simulink model "sim_quadrotor_16b"  (R2016b)
settings: Solver=ode4  StartTime=0.0  StopTime=20  FixedStep=0.0001  RelTol=1e-3
undefined symbols (not defined in the file or in its folder): Ag_phi_rad, Ag_psi_rad, Ag_theta_rad, AgVel_p_radPerScnd, AgVel_q_radPerScnd, AgVel_r_radPerScnd, Ap, Aq, Ar, Az, Bp, Bq, Br, Bz, C, D, par, Pos_z_mtr, V_w_mtrPerScnd
settings Model: Creator=Nu  LastModifiedBy=Nu

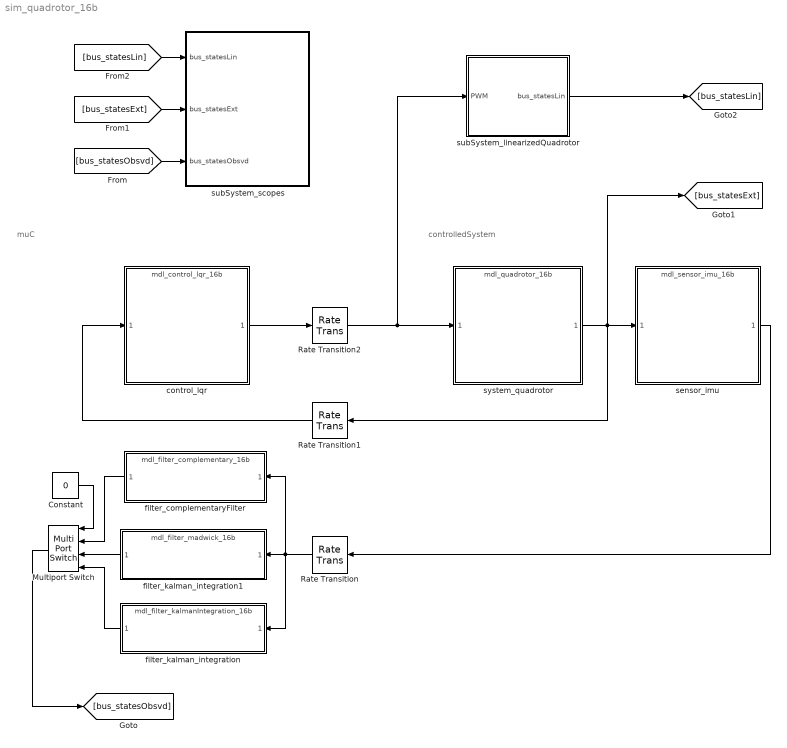
== system sim_quadrotor_16b ==
  note: controlledSystem
  note: muC
  Constant : Constant  Value=0
  Multiport Switch : MultiPortSwitch  DataPortOrder=Zero-based contiguous
  Rate Transition : RateTransition  OutPortSampleTime=filterKalman_par.T
  Rate Transition1 : RateTransition
  Rate Transition2 : RateTransition
  control_lqr : ModelReference  ModelNameDialog=mdl_control_lqr_16b.slx  SimulationMode=Normal  ModelReferenceVersion=1.230
  filter_complementaryFilter : ModelReference  ModelNameDialog=mdl_filter_complementary_16b.slx  SimulationMode=Normal  ModelReferenceVersion=1.30
  filter_kalman_integration : ModelReference  ModelNameDialog=mdl_filter_kalmanIntegration_16b.slx  SimulationMode=Normal  ModelReferenceVersion=1.24
  filter_kalman_integration1 : ModelReference  ModelNameDialog=mdl_filter_madwick_16b.slx  SimulationMode=Normal  ModelReferenceVersion=1.24
  sensor_imu : ModelReference  ModelNameDialog=mdl_sensor_imu_16b.slx  SimulationMode=Normal  ModelReferenceVersion=1.231
  subSystem_linearizedQuadrotor : Subsystem
  subSystem_scopes : Subsystem
  system_quadrotor : ModelReference  ModelNameDialog=mdl_quadrotor_16b.slx  SimulationMode=Normal  ModelReferenceVersion=1.231
  wires:
  system_quadrotor/1 -> Rate Transition1/1, sensor_imu/1, [bus_statesExt]
  control_lqr/1 -> Rate Transition2/1
  sensor_imu/1 -> Rate Transition/1
  [bus_statesObsvd] -> subSystem_scopes/3(bus_statesObsvd)
  [bus_statesExt] -> subSystem_scopes/2(bus_statesExt)
  [bus_statesLin] -> subSystem_scopes/1(bus_statesLin)
  subSystem_linearizedQuadrotor/1(bus_statesLin) -> [bus_statesLin]
  Rate Transition2/1 -> system_quadrotor/1, subSystem_linearizedQuadrotor/1(PWM)
  Multiport Switch/1 -> [bus_statesObsvd]
  Rate Transition/1 -> filter_kalman_integration1/1, filter_complementaryFilter/1, filter_kalman_integration/1
  Rate Transition1/1 -> control_lqr/1
  filter_complementaryFilter/1 -> Multiport Switch/2
  filter_kalman_integration/1 -> Multiport Switch/4
  filter_kalman_integration1/1 -> Multiport Switch/3
  Constant/1 -> Multiport Switch/1

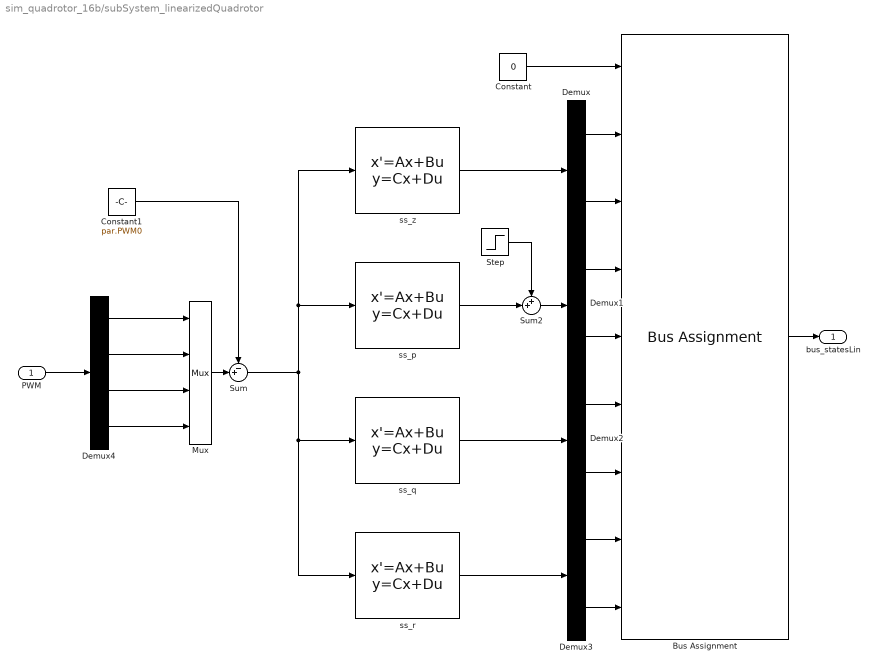
== system sim_quadrotor_16b/subSystem_linearizedQuadrotor ==
  PWM : Inport
  Bus Assignment : BusAssignment  AssignedSignals=Pos_z_mtr,V_w_mtrPerScnd,Ag_phi_rad,AgVel_p_radPerScnd,Ag_theta_rad,AgVel_q_radPerScnd,Ag_psi_rad,AgVel_r_radPerScnd
  Constant : Constant  Value=0  OutDataTypeStr=Bus: mdl_statesExt
  Constant1 : Constant  Value=par.PWM0
  Demux{,1..3} (4 alike) : Demux  Outputs=2
  Demux4 : Demux
  Mux : Mux
  Step : Step  Time=5  Before=[0 0]  After=[2*pi/180 0 ]  SampleTime=0
  Sum : Sum  Inputs=-+|
  Sum2 : Sum  Inputs=++|
  ss_p : StateSpace  A=Ap  B=Bp  C=C  D=D  X0=0
  ss_q : StateSpace  A=Aq  B=Bq  C=C  D=D  X0=0
  ss_r : StateSpace  A=Ar  B=Br  C=C  D=D  X0=0
  ss_z : StateSpace  A=Az  B=Bz  C=C  D=D  X0=0
  bus_statesLin : Outport
  wires:
  Demux4/1 -> Mux/1
  Demux4/4 -> Mux/4
  Demux4/3 -> Mux/3
  Demux4/2 -> Mux/2
  Sum/1 -> ss_q/1, ss_r/1, ss_p/1, ss_z/1
  Bus Assignment/1 -> bus_statesLin/1
  Constant/1 -> Bus Assignment/1
  Demux/1 -> Bus Assignment/2
  Demux/2 -> Bus Assignment/3
  Demux1/1 -> Bus Assignment/4
  Demux1/2 -> Bus Assignment/5
  Demux2/1 -> Bus Assignment/6
  Demux2/2 -> Bus Assignment/7
  Demux3/1 -> Bus Assignment/8
  Demux3/2 -> Bus Assignment/9
  ss_p/1 -> Sum2/2
  ss_q/1 -> Demux2/1
  ss_r/1 -> Demux3/1
  ss_z/1 -> Demux/1
  Mux/1 -> Sum/2
  Constant1/1 -> Sum/1
  Step/1 -> Sum2/1
  Sum2/1 -> Demux1/1
  PWM/1 -> Demux4/1

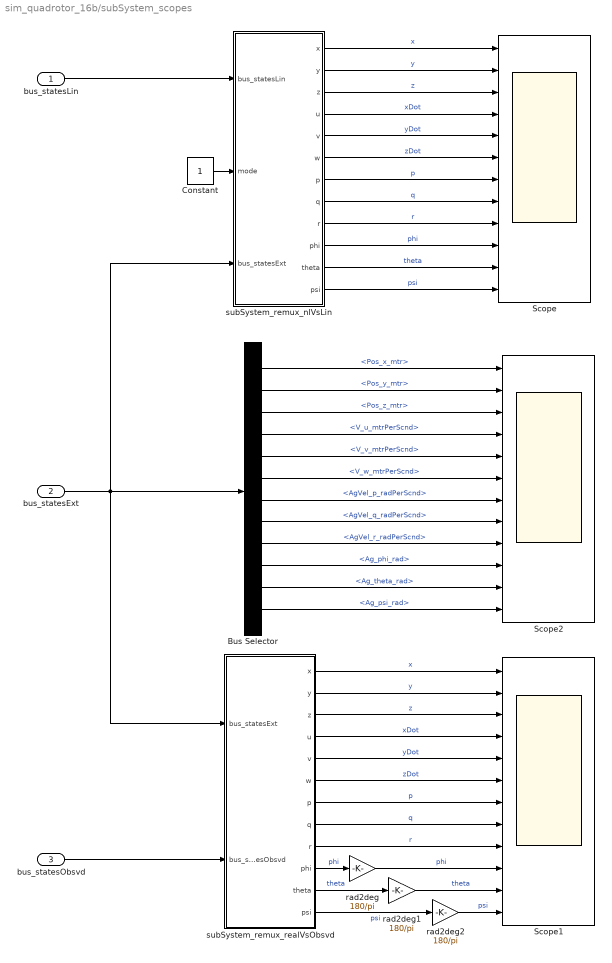
== system sim_quadrotor_16b/subSystem_scopes ==
  bus_statesLin : Inport
  bus_statesExt : Inport  Port=2
  bus_statesObsvd : Inport  Port=3
  Bus Selector : BusSelector  OutputSignals=Pos_x_mtr,Pos_y_mtr,Pos_z_mtr,V_u_mtrPerScnd,V_v_mtrPerScnd,V_w_mtrPerScnd,AgVel_p_radPerScnd,AgVel_q_radPerScnd,AgVel_r_radPerScnd,Ag_phi_rad,Ag_theta_rad,Ag_psi_rad
  Constant : Constant
  Scope : Scope  NumInputPorts=12
  Scope1 : Scope  NumInputPorts=12
  Scope2 : Scope  NumInputPorts=12
  rad2deg : Gain  Gain=180/pi
  rad2deg1 : Gain  Gain=180/pi
  rad2deg2 : Gain  Gain=180/pi
  subSystem_remux_nlVsLin : Subsystem
  subSystem_remux_realVsObsvd : Subsystem
  wires:
  bus_statesLin/1 -> subSystem_remux_nlVsLin/1(bus_statesLin)
  subSystem_remux_nlVsLin/1(x) -> Scope/1  "x"
  subSystem_remux_nlVsLin/2(y) -> Scope/2  "y"
  subSystem_remux_nlVsLin/3(z) -> Scope/3  "z"
  subSystem_remux_nlVsLin/4(u) -> Scope/4  "xDot"
  subSystem_remux_nlVsLin/5(v) -> Scope/5  "yDot"
  subSystem_remux_nlVsLin/6(w) -> Scope/6  "zDot"
  subSystem_remux_nlVsLin/7(p) -> Scope/7  "p"
  subSystem_remux_nlVsLin/8(q) -> Scope/8  "q"
  subSystem_remux_nlVsLin/9(r) -> Scope/9  "r"
  subSystem_remux_nlVsLin/10(phi) -> Scope/10  "phi"
  subSystem_remux_nlVsLin/11(theta) -> Scope/11  "theta"
  subSystem_remux_nlVsLin/12(psi) -> Scope/12  "psi"
  subSystem_remux_realVsObsvd/1(x) -> Scope1/1  "x"
  subSystem_remux_realVsObsvd/2(y) -> Scope1/2  "y"
  subSystem_remux_realVsObsvd/3(z) -> Scope1/3  "z"
  subSystem_remux_realVsObsvd/4(u) -> Scope1/4  "xDot"
  subSystem_remux_realVsObsvd/5(v) -> Scope1/5  "yDot"
  subSystem_remux_realVsObsvd/6(w) -> Scope1/6  "zDot"
  subSystem_remux_realVsObsvd/7(p) -> Scope1/7  "p"
  subSystem_remux_realVsObsvd/8(q) -> Scope1/8  "q"
  subSystem_remux_realVsObsvd/9(r) -> Scope1/9  "r"
  subSystem_remux_realVsObsvd/10(phi) -> rad2deg/1  "phi"
  subSystem_remux_realVsObsvd/11(theta) -> rad2deg1/1  "theta"
  subSystem_remux_realVsObsvd/12(psi) -> rad2deg2/1  "psi"
  Constant/1 -> subSystem_remux_nlVsLin/2(mode)
  bus_statesExt/1 -> subSystem_remux_nlVsLin/3(bus_statesExt), Bus Selector/1, subSystem_remux_realVsObsvd/1(bus_statesExt)
  bus_statesObsvd/1 -> subSystem_remux_realVsObsvd/2(bus_statesObsvd)
  rad2deg/1 -> Scope1/10  "phi"
  rad2deg1/1 -> Scope1/11  "theta"
  rad2deg2/1 -> Scope1/12  "psi"
  Bus Selector/1 -> Scope2/1  "<Pos_x_mtr>"
  Bus Selector/2 -> Scope2/2  "<Pos_y_mtr>"
  Bus Selector/3 -> Scope2/3  "<Pos_z_mtr>"
  Bus Selector/4 -> Scope2/4  "<V_u_mtrPerScnd>"
  Bus Selector/5 -> Scope2/5  "<V_v_mtrPerScnd>"
  Bus Selector/6 -> Scope2/6  "<V_w_mtrPerScnd>"
  Bus Selector/7 -> Scope2/7  "<AgVel_p_radPerScnd>"
  Bus Selector/8 -> Scope2/8  "<AgVel_q_radPerScnd>"
  Bus Selector/9 -> Scope2/9  "<AgVel_r_radPerScnd>"
  Bus Selector/10 -> Scope2/10  "<Ag_phi_rad>"
  Bus Selector/11 -> Scope2/11  "<Ag_theta_rad>"
  Bus Selector/12 -> Scope2/12  "<Ag_psi_rad>"

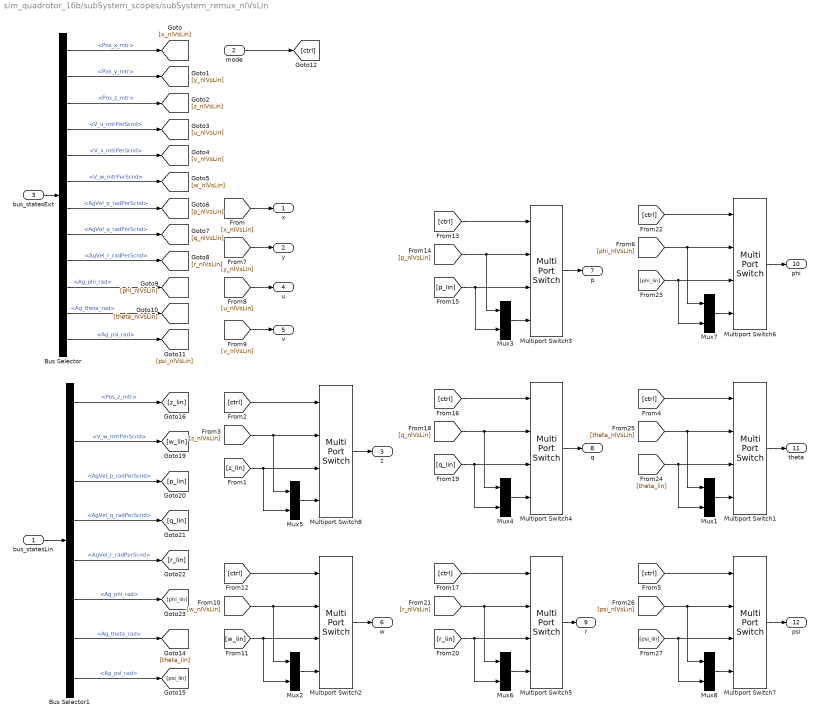
== system sim_quadrotor_16b/subSystem_scopes/subSystem_remux_nlVsLin ==
  bus_statesLin : Inport
  mode : Inport  Port=2
  bus_statesExt : Inport  Port=3
  Bus Selector : BusSelector  OutputSignals=Pos_x_mtr,Pos_y_mtr,Pos_z_mtr,V_u_mtrPerScnd,V_v_mtrPerScnd,V_w_mtrPerScnd,AgVel_p_radPerScnd,AgVel_q_radPerScnd,AgVel_r_radPerScnd,Ag_phi_rad,Ag_theta_rad,Ag_psi_rad
  Bus Selector1 : BusSelector  OutputSignals=Pos_z_mtr,V_w_mtrPerScnd,AgVel_p_radPerScnd,AgVel_q_radPerScnd,AgVel_r_radPerScnd,Ag_phi_rad,Ag_theta_rad,Ag_psi_rad
  Multiport Switch{1..8} (8 alike) : MultiPortSwitch
  Mux{1..8} (8 alike) : Mux  Inputs=2
  x : Outport
  y : Outport  Port=2
  z : Outport  Port=3
  u : Outport  Port=4
  v : Outport  Port=5
  w : Outport  Port=6
  p : Outport  Port=7
  q : Outport  Port=8
  r : Outport  Port=9
  phi : Outport  Port=10
  theta : Outport  Port=11
  psi : Outport  Port=12
  wires:
  Bus Selector/1 -> [x_nlVsLin]  "<Pos_x_mtr>"
  bus_statesExt/1 -> Bus Selector/1
  bus_statesLin/1 -> Bus Selector1/1
  Multiport Switch8/1 -> z/1
  Multiport Switch2/1 -> w/1
  Multiport Switch3/1 -> p/1
  Multiport Switch4/1 -> q/1
  Multiport Switch5/1 -> r/1
  Bus Selector/3 -> [z_nlVsLin]  "<Pos_z_mtr>"
  Bus Selector/2 -> [y_nlVsLin]  "<Pos_y_mtr>"
  Bus Selector/4 -> [u_nlVsLin]  "<V_u_mtrPerScnd>"
  Bus Selector/5 -> [v_nlVsLin]  "<V_v_mtrPerScnd>"
  Bus Selector/6 -> [w_nlVsLin]  "<V_w_mtrPerScnd>"
  Bus Selector/7 -> [p_nlVsLin]  "<AgVel_p_radPerScnd>"
  Bus Selector/8 -> [q_nlVsLin]  "<AgVel_q_radPerScnd>"
  Bus Selector/12 -> [psi_nlVsLin]  "<Ag_psi_rad>"
  Bus Selector/11 -> [theta_nlVsLin]  "<Ag_theta_rad>"
  Bus Selector/10 -> [phi_nlVsLin]  "<Ag_phi_rad>"
  Bus Selector/9 -> [r_nlVsLin]  "<AgVel_r_radPerScnd>"
  Bus Selector1/1 -> [z_lin]  "<Pos_z_mtr>"
  Bus Selector1/2 -> [w_lin]  "<V_w_mtrPerScnd>"
  Bus Selector1/3 -> [p_lin]  "<AgVel_p_radPerScnd>"
  Bus Selector1/4 -> [q_lin]  "<AgVel_q_radPerScnd>"
  Bus Selector1/5 -> [r_lin]  "<AgVel_r_radPerScnd>"
  Bus Selector1/6 -> [phi_lin]  "<Ag_phi_rad>"
  Bus Selector1/7 -> [theta_lin]  "<Ag_theta_rad>"
  Bus Selector1/8 -> [psi_lin]  "<Ag_psi_rad>"
  Mux5/1 -> Multiport Switch8/4
  [z_lin] -> Mux5/2, Multiport Switch8/3
  [x_nlVsLin] -> x/1
  mode/1 -> [ctrl]
  [ctrl] -> Multiport Switch8/1
  [z_nlVsLin] -> Mux5/1, Multiport Switch8/2
  [y_nlVsLin] -> y/1
  [u_nlVsLin] -> u/1
  [v_nlVsLin] -> v/1
  Mux2/1 -> Multiport Switch2/4
  [w_lin] -> Mux2/2, Multiport Switch2/3
  [ctrl] -> Multiport Switch2/1
  [w_nlVsLin] -> Multiport Switch2/2, Mux2/1
  Mux3/1 -> Multiport Switch3/4
  [p_lin] -> Multiport Switch3/3, Mux3/2
  [ctrl] -> Multiport Switch3/1
  [p_nlVsLin] -> Multiport Switch3/2, Mux3/1
  Mux4/1 -> Multiport Switch4/4
  [q_lin] -> Mux4/2, Multiport Switch4/3
  [ctrl] -> Multiport Switch4/1
  [q_nlVsLin] -> Multiport Switch4/2, Mux4/1
  Mux6/1 -> Multiport Switch5/4
  [r_lin] -> Mux6/2, Multiport Switch5/3
  [ctrl] -> Multiport Switch5/1
  [r_nlVsLin] -> Multiport Switch5/2, Mux6/1
  Mux7/1 -> Multiport Switch6/4
  [phi_lin] -> Mux7/2, Multiport Switch6/3
  [ctrl] -> Multiport Switch6/1
  [phi_nlVsLin] -> Multiport Switch6/2, Mux7/1
  Multiport Switch6/1 -> phi/1
  Mux1/1 -> Multiport Switch1/4
  [theta_lin] -> Mux1/2, Multiport Switch1/3
  [ctrl] -> Multiport Switch1/1
  [theta_nlVsLin] -> Multiport Switch1/2, Mux1/1
  Multiport Switch1/1 -> theta/1
  Mux8/1 -> Multiport Switch7/4
  [psi_lin] -> Mux8/2, Multiport Switch7/3
  [ctrl] -> Multiport Switch7/1
  [psi_nlVsLin] -> Multiport Switch7/2, Mux8/1
  Multiport Switch7/1 -> psi/1

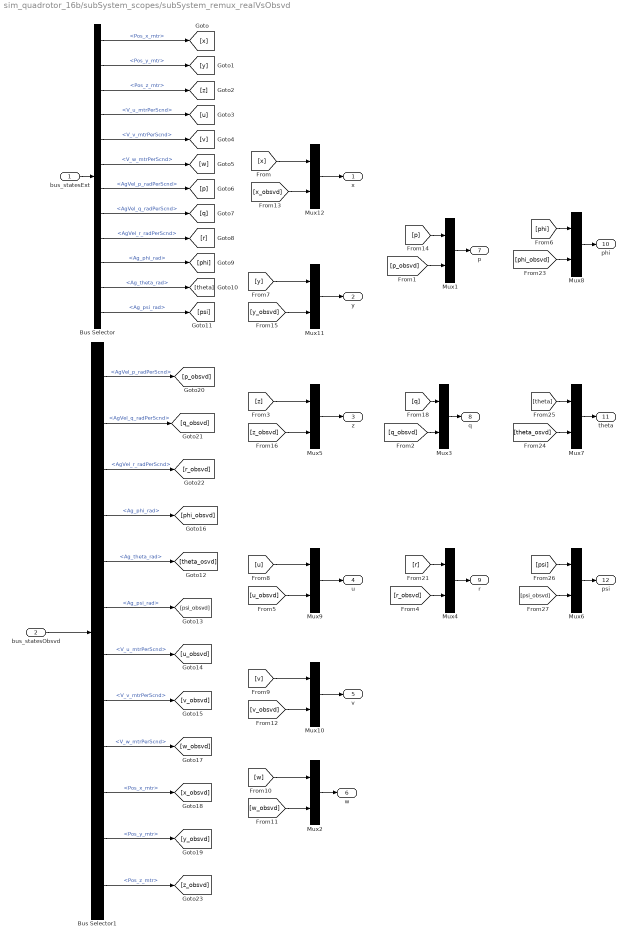
== system sim_quadrotor_16b/subSystem_scopes/subSystem_remux_realVsObsvd ==
  bus_statesExt : Inport
  bus_statesObsvd : Inport  Port=2
  Bus Selector : BusSelector  OutputSignals=Pos_x_mtr,Pos_y_mtr,Pos_z_mtr,V_u_mtrPerScnd,V_v_mtrPerScnd,V_w_mtrPerScnd,AgVel_p_radPerScnd,AgVel_q_radPerScnd,AgVel_r_radPerScnd,Ag_phi_rad,Ag_theta_rad,Ag_psi_rad
  Bus Selector1 : BusSelector  OutputSignals=AgVel_p_radPerScnd,AgVel_q_radPerScnd,AgVel_r_radPerScnd,Ag_phi_rad,Ag_theta_rad,Ag_psi_rad,V_u_mtrPerScnd,V_v_mtrPerScnd,V_w_mtrPerScnd,Pos_x_mtr,Pos_y_mtr,Pos_z_mtr
  Mux{1..12} (12 alike) : Mux  Inputs=2
  x : Outport
  y : Outport  Port=2
  z : Outport  Port=3
  u : Outport  Port=4
  v : Outport  Port=5
  w : Outport  Port=6
  p : Outport  Port=7
  q : Outport  Port=8
  r : Outport  Port=9
  phi : Outport  Port=10
  theta : Outport  Port=11
  psi : Outport  Port=12
  wires:
  [z] -> Mux5/1
  [z_obsvd] -> Mux5/2
  Bus Selector1/3 -> [r_obsvd]  "<AgVel_r_radPerScnd>"
  Bus Selector1/2 -> [q_obsvd]  "<AgVel_q_radPerScnd>"
  Bus Selector1/1 -> [p_obsvd]  "<AgVel_p_radPerScnd>"
  Bus Selector/9 -> [r]  "<AgVel_r_radPerScnd>"
  Bus Selector/10 -> [phi]  "<Ag_phi_rad>"
  Bus Selector/11 -> [theta]  "<Ag_theta_rad>"
  Bus Selector/12 -> [psi]  "<Ag_psi_rad>"
  Bus Selector/8 -> [q]  "<AgVel_q_radPerScnd>"
  Bus Selector/7 -> [p]  "<AgVel_p_radPerScnd>"
  Bus Selector/6 -> [w]  "<V_w_mtrPerScnd>"
  Bus Selector/5 -> [v]  "<V_v_mtrPerScnd>"
  Bus Selector/4 -> [u]  "<V_u_mtrPerScnd>"
  Bus Selector/2 -> [y]  "<Pos_y_mtr>"
  Bus Selector/3 -> [z]  "<Pos_z_mtr>"
  Mux2/1 -> w/1
  Mux5/1 -> z/1
  bus_statesObsvd/1 -> Bus Selector1/1
  bus_statesExt/1 -> Bus Selector/1
  Bus Selector/1 -> [x]  "<Pos_x_mtr>"
  [w] -> Mux2/1
  [w_obsvd] -> Mux2/2
  [p] -> Mux1/1
  [p_obsvd] -> Mux1/2
  [q] -> Mux3/1
  [q_obsvd] -> Mux3/2
  [r] -> Mux4/1
  [r_obsvd] -> Mux4/2
  [psi] -> Mux6/1
  [psi_obsvd] -> Mux6/2
  [theta] -> Mux7/1
  [theta_osvd] -> Mux7/2
  [phi] -> Mux8/1
  [phi_obsvd] -> Mux8/2
  Mux1/1 -> p/1
  Mux3/1 -> q/1
  Mux4/1 -> r/1
  Mux6/1 -> psi/1
  Mux7/1 -> theta/1
  Mux8/1 -> phi/1
  Bus Selector1/5 -> [theta_osvd]  "<Ag_theta_rad>"
  Bus Selector1/6 -> [psi_obsvd]  "<Ag_psi_rad>"
  Bus Selector1/4 -> [phi_obsvd]  "<Ag_phi_rad>"
  Bus Selector1/7 -> [u_obsvd]  "<V_u_mtrPerScnd>"
  Bus Selector1/8 -> [v_obsvd]  "<V_v_mtrPerScnd>"
  Bus Selector1/9 -> [w_obsvd]  "<V_w_mtrPerScnd>"
  Mux9/1 -> u/1
  [u] -> Mux9/1
  [u_obsvd] -> Mux9/2
  Mux10/1 -> v/1
  [v] -> Mux10/1
  [v_obsvd] -> Mux10/2
  Bus Selector1/12 -> [z_obsvd]  "<Pos_z_mtr>"
  Bus Selector1/11 -> [y_obsvd]  "<Pos_y_mtr>"
  Bus Selector1/10 -> [x_obsvd]  "<Pos_x_mtr>"
  [y_obsvd] -> Mux11/2
  [y] -> Mux11/1
  Mux11/1 -> y/1
  [x_obsvd] -> Mux12/2
  [x] -> Mux12/1
  Mux12/1 -> x/1
